simulink model "EOM_ECEF_6DOF"  (R2023a)
settings: Solver=ode4  StartTime=0.0  StopTime=tf  FixedStep=dt  RelTol=1e-3
values from neighbouring files (symbols this model uses):
  F = [0, 0, 0]    [verifyEOM.m]
  M = [0, 0, 0]    [verifyEOM.m]
  mass = 5000    [verifyEOM.m]
  testRotational = 0    [verifyEOM.m]
  testTranslational = 1    [verifyEOM.m]
undefined symbols (not defined in the file or in its folder): Earth, WGS84
libraries: aerolib6dof2 x1, dspsigattribs x1
settings Model: Creator=cmonti  LastModifiedBy=cmonti
settings DataIOCC: SaveOutput=off  SignalLogging=off  DSMLogging=off  SaveTime=off  ReturnWorkspaceOutputs=off

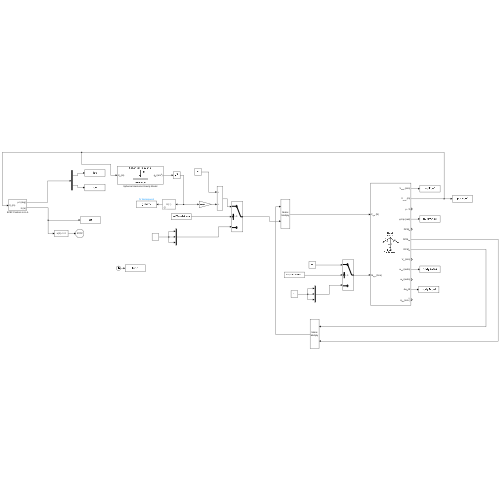
[thumbnail: Simulink's stored preview of the top-level diagram]
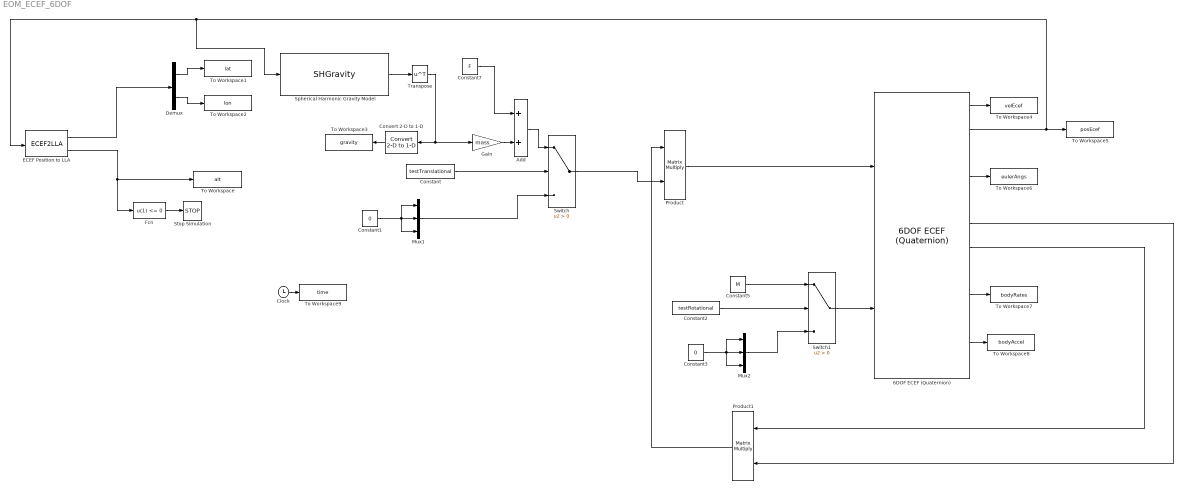
== system EOM_ECEF_6DOF ==
  6DOF ECEF (Quaternion) : aerolib6dof2/6DOF ECEF (Quaternion)  units=Metric (MKS)  mtype=Fixed  xg_0=[0 0 1e3]  Vm_0=[0 0 0]  eul_0=[0 0 0]  pm_0=[0 0 0]  mass_0=mass  mass_e=0.5  mass_f=2.0  inertia=[50, 10, 10; 10, 100, 15; 10, 15, 120]  inertia_e=eye(3)  inertia_f=2*eye(3)  vre_flag=on  abi_flag=off  ptype=Earth (WGS84)  R=6378137  F=1/298.257223563  w_E=7292115e-11  angle_in=Internal  LG0=0  quat_statename=''  pm_statename=''  Vm_statename=''  posECEF_statename=''  posECI_statename=''  LG_statename=''  mass_statename=''
  Add : Sum
  Clock : Clock
  Constant : Constant  Value=testTranslational
  Constant1 : Constant  Value=0
  Constant2 : Constant  Value=testRotational
  Constant3 : Constant  Value=0
  Constant5 : Constant  Value=M
  Constant7 : Constant  Value=F
  Convert 2-D to 1-D : dspsigattribs/Convert 2-D to 1-D
  Demux : Demux  Outputs=2
  ECEF Position to LLA : ECEF2LLA
  Fcn : Fcn  Expr=u(1) <= 0
  Gain : Gain  Gain=mass
  Mux1 : Mux  Inputs=3
  Mux2 : Mux  Inputs=3
  Product : Product  Multiplication=Matrix(*)
  Product1 : Product  Multiplication=Matrix(*)
  Spherical Harmonic Gravity Model : SHGravity
  Stop Simulation : Stop
  Switch : Switch  Criteria=u2 > Threshold  SaturateOnIntegerOverflow=off  InputSameDT=off
  Switch1 : Switch  Criteria=u2 > Threshold  SaturateOnIntegerOverflow=off  InputSameDT=off
  To Workspace : ToWorkspace  VariableName=alt  SampleTime=-1
  To Workspace1 : ToWorkspace  VariableName=lat  SampleTime=-1
  To Workspace2 : ToWorkspace  VariableName=lon  SampleTime=-1
  To Workspace3 : ToWorkspace  VariableName=gravity  SampleTime=-1
  To Workspace4 : ToWorkspace  VariableName=velEcef  SampleTime=-1
  To Workspace5 : ToWorkspace  VariableName=posEcef  SampleTime=-1
  To Workspace6 : ToWorkspace  VariableName=eulerAngs  SampleTime=-1
  To Workspace7 : ToWorkspace  VariableName=bodyRates  SampleTime=-1
  To Workspace8 : ToWorkspace  VariableName=bodyAccel  SampleTime=-1
  To Workspace9 : ToWorkspace  VariableName=time  SampleTime=-1
  Transpose : Math  Operator=transpose
  wires:
  ECEF Position to LLA/1 -> Demux/1
  6DOF ECEF (Quaternion)/2 -> To Workspace5/1, ECEF Position to LLA/1, Spherical Harmonic Gravity Model/1
  Constant/1 -> Switch/2
  Constant1/1 -> Mux1/3, Mux1/1, Mux1/2
  Mux1/1 -> Switch/3
  Mux2/1 -> Switch1/3
  Constant3/1 -> Mux2/2, Mux2/1, Mux2/3
  Constant2/1 -> Switch1/2
  Switch1/1 -> 6DOF ECEF (Quaternion)/2
  ECEF Position to LLA/2 -> Fcn/1, To Workspace/1
  Fcn/1 -> Stop Simulation/1
  Demux/2 -> To Workspace2/1
  Demux/1 -> To Workspace1/1
  Add/1 -> Switch/1
  Constant7/1 -> Add/1
  Constant5/1 -> Switch1/1
  6DOF ECEF (Quaternion)/1 -> To Workspace4/1
  6DOF ECEF (Quaternion)/4 -> To Workspace6/1
  6DOF ECEF (Quaternion)/11 -> To Workspace8/1
  6DOF ECEF (Quaternion)/9 -> To Workspace7/1
  Clock/1 -> To Workspace9/1
  Switch/1 -> Product/2
  Product/1 -> 6DOF ECEF (Quaternion)/1
  Gain/1 -> Add/2
  Spherical Harmonic Gravity Model/1 -> Transpose/1
  Transpose/1 -> Gain/1, Convert 2-D to 1-D/1
  Convert 2-D to 1-D/1 -> To Workspace3/1
  Product1/1 -> Product/1
  6DOF ECEF (Quaternion)/7 -> Product1/1
  6DOF ECEF (Quaternion)/6 -> Product1/2
